simulink model "consensus"  (Simulink 7.4)
settings: Solver=ode45  StartTime=0.0  StopTime=10.0  RelTol=1e-3
settings Model: Creator=chepeadan  LastModifiedBy=francisco

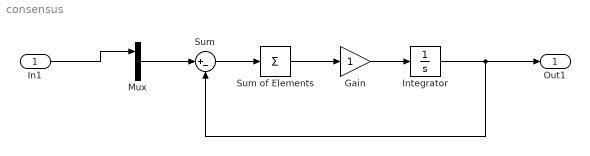
== system consensus ==
  In1 : Inport
  Gain : Gain  ParameterDataType=fixdt(1, 16)  ParameterScaling=2^0  OutDataType=fixdt(1, 16)  OutScaling=2^0
  Integrator : Integrator  InitialCondition=100*(rand()-0.5)
  Mux : Mux  Inputs=2
  Sum : Sum  Inputs=|+-  OutDataType=fixdt(1, 16)  OutScaling=2^0
  Sum of Elements : Sum  Inputs=+  OutDataType=fixdt(1, 16)  OutScaling=2^-10
  Out1 : Outport
  wires:
  In1/1 -> Mux/1
  Mux/1 -> Sum/1
  Sum/1 -> Sum of Elements/1
  Sum of Elements/1 -> Gain/1
  Gain/1 -> Integrator/1
  Integrator/1 -> Out1/1, Sum/2
